simulink model "Adapted_AD9856"  (Simulink 7.6)
settings: Solver=VariableStepDiscrete  StartTime=0.0  StopTime=20000 * SampleTime  RelTol=1e-3
PreLoadFcn:
  | setup_Adapted_AD9856;
InitFcn:
  | setup_Adapted_AD9856;
  | %% DSPBuilder Start
  | alt_dspbuilder_update_model(bdroot)
  | %% DSPBuilder End
values from neighbouring files (symbols this model uses):
  ChanCount = 2    [setup_Adapted_AD9856.m]
  Period = ClockRate / SampleRate    (= 80)    [setup_Adapted_AD9856.m]
  SampleRate = ' num2str(SampleRate) '    [setup_Adapted_AD9856.m]
  SampleTime = ' num2str(SampleTime) ';'])    [setup_Adapted_AD9856.m]
undefined symbols (not defined in the file or in its folder): dpoly, dspba_ChannelInVis, dspba_ChannelOutVis, dspba_internal_get_channel_ports, firhalfband, get, value
libraries: DSPBABase x20, DSPBAPrim x20, allblocks_alteradspbuilder2 x13, simulink x12, DSPBAFilters x5, dspsigops x2, dspsnks4 x2, DSPBAWaveformSynth x1
settings Model: Creator=lkong  LastModifiedBy=akarapet
settings OptimizationCC: InitFltsAndDblsToZero=on
settings DebuggingCC: StrictBusMsg=Warning

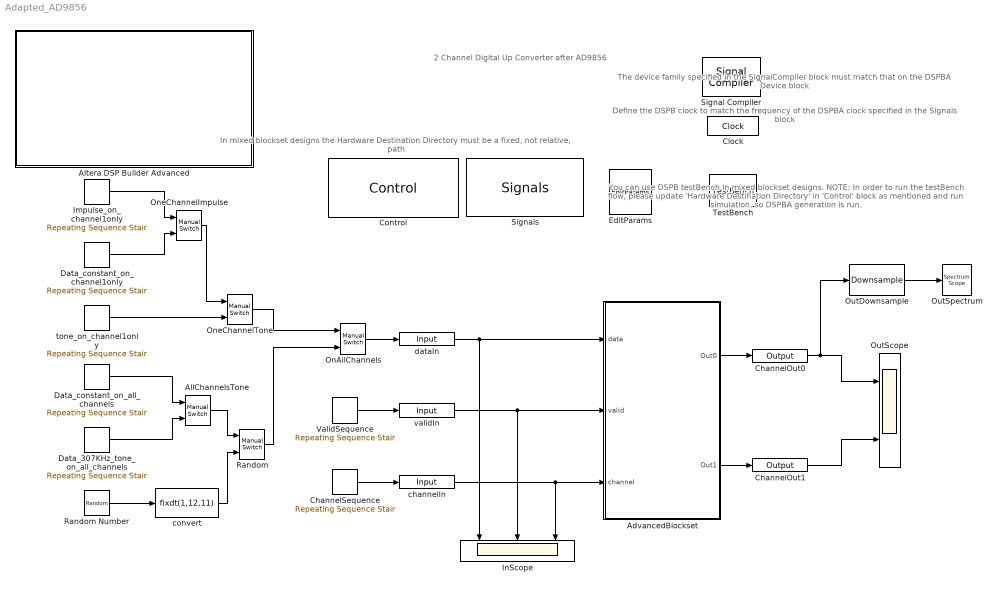
== system Adapted_AD9856 ==
  note: 2 Channel Digital Up Converter after AD9856
  note: In mixed blockset designs the Hardware Destination
      | Directory must be a fixed, not relative, path
  note: Define the DSPB clock to match the frequency of
      | the DSPBA clock specified in the Signals block
  note: You can use DSPB testBench in mixed blockset designs.
      |
      | NOTE: In order to run the testBench flow,  please update
      | 'Hardware Destination Directory' in 'Control' block as mentioned
      | and run simulation, so DSPBA generation is run.
  note: The device family specified in the SignalCompiler
      | block must match that on the DSPBA Device block
  AdvancedBlockset : Subsystem
  AllChannelsTone : simulink/Signal Routing/Manual Switch  SystemSampleTime=-1  sw=0  action=0  varsize=off
  Altera DSP Builder Advanced : Subsystem
      settings: OpenFcn=web('http://www.altera.com', '-new');
      mask Type: DSP Builder Advanced Blockset Ignored Block
      mask Display: image(imread('alteralogo.tif'));
  ChannelOut0 : allblocks_alteradspbuilder2/Output  iofile=/data/akarapet/qshell_linux64_test/p4/dsp_builder/dsp_builder2/Documentation/DesignExamples/Demos/CombinedBlockset/demo_adapted_ad9856/tb_Adapted_AD9856/Adapted%5FAD9856_ChannelOut0.capture  BusType=Signed Fractional  bwl=1  bwr=15  externalType=Inferred  PORTTYPE=Output  allowFloatingPointOverride=on  logOutputs=off
  ChannelOut1 : allblocks_alteradspbuilder2/Output  iofile=/data/akarapet/qshell_linux64_test/p4/dsp_builder/dsp_builder2/Documentation/DesignExamples/Demos/CombinedBlockset/demo_adapted_ad9856/tb_Adapted_AD9856/Adapted%5FAD9856_ChannelOut1.capture  BusType=Signed Fractional  bwl=1  bwr=15  externalType=Inferred  PORTTYPE=Output  allowFloatingPointOverride=on  logOutputs=off
  ChannelSequence : simulink/Sources/Repeating Sequence Stair  SystemSampleTime=-1  OutValues=[[0:ChanCount-1] zeros(1,Period-ChanCount)].'  tsamp=SampleTime  OutMin=[]  OutMax=[]  OutDataTypeStr=fixdt(0,8,0)  OutputDataTypeScalingMode=Specify via dialog  OutDataType=ufix(8)  ConRadixGroup=Use specified scaling  OutScaling=2^-0
  Clock : allblocks_alteradspbuilder2/Clock  ClockPeriod=50  ClockPeriodUnit=ns  SampleTime=1  ResetLatency=0  ResetRegisterCascadeDepth=0  SimulationStartCycle=5  PhaseOffset=0  Reset=aclr  ResetType=Active Low  Export=off
  Control : DSPBABase/Control  generate=on  destination=.  language=VHDL  autotestbench=on  signaldepth=2  coveragetestbench=on  logs=off  spacewidth=2  spacenum=1  addrwidth=12  datawidth=32  dataendian=Big Endian  hierarchicalnames=on  ramThresholdBits=-1  distRamThresholdBits=-1  mlabThresholdBits=-1  hardMultiplierThresholdLuts=-1  version=20090407  errorOnChanMismatch=1  errorOnGPIOMismatch=0  importModelsimResults=0
  Data_307KHz_tone_on_all_channels : simulink/Sources/Repeating Sequence Stair  SystemSampleTime=-1  OutValues="floor([(ChanCount:-1:1)/ChanCount * 1 zeros(1, Period-ChanCount) (ChanCount:-1:1)/ChanCount  * 0 zeros(1, Period-ChanCount) (ChanCount:-1:1)/ChanCount * -1 zeros(1, Period-ChanCount) (ChanCount:-1:1)/ChanCount * 0 zeros(1, Period-ChanCount) ]*1412) / 2^11"  tsamp=SampleTime  OutMin=[]  OutMax=[]  OutDataTypeStr=fixdt(1,12,11)  OutputDataTypeScalingMode=Specify via dialog  OutDataType=sfix(12)  ConRadixGroup=Use specified scaling  OutScaling=2^-11
  Data_constant_on_all_channels : simulink/Sources/Repeating Sequence Stair  SystemSampleTime=-1  OutValues=floor([(ChanCount:-1:1)/ChanCount zeros(1, Period-ChanCount)] * 1412) / 2^11  tsamp=SampleTime  OutMin=[]  OutMax=[]  OutDataTypeStr=fixdt(1,12,11)  OutputDataTypeScalingMode=Specify via dialog  OutDataType=sfix(12)  ConRadixGroup=Use specified scaling  OutScaling=2^-11
  Data_constant_on_channel1only : simulink/Sources/Repeating Sequence Stair  SystemSampleTime=-1  OutValues="[ones(1, 1)  * 1 zeros(1, 199) ]*(1412 / 2^11)"  tsamp=SampleTime  OutMin=[]  OutMax=[]  OutDataTypeStr=fixdt(1,12,11)  OutputDataTypeScalingMode=Specify via dialog  OutDataType=sfix(12)  ConRadixGroup=Use specified scaling  OutScaling=2^-11
  EditParams : DSPBABase/EditParams  SystemSampleTime=-1  version=20090407
  Impulse_on_channel1only : simulink/Sources/Repeating Sequence Stair  SystemSampleTime=-1  OutValues="[ones(1, 1)  * 1 zeros(1, 19900) ]*(1000 / 2^11)"  tsamp=SampleTime  OutMin=[]  OutMax=[]  OutDataTypeStr=fixdt(1,12,11)  OutputDataTypeScalingMode=Specify via dialog  OutDataType=sfix(12)  ConRadixGroup=Use specified scaling  OutScaling=2^-11
  InScope : Scope  NumInputPorts=3
      settings: TimeRange=10000  YMin=-1~-1.5~-1.5  YMax=1~1.5~1.5  SaveName=ScopeData5
  OnAllChannels : simulink/Signal Routing/Manual Switch  SystemSampleTime=-1  sw=0  action=0  varsize=off
  OneChannelImpulse : simulink/Signal Routing/Manual Switch  SystemSampleTime=-1  sw=1  action=0  varsize=off
  OneChannelTone : simulink/Signal Routing/Manual Switch  SystemSampleTime=-1  sw=1  action=0  varsize=off
  OutDownsample : dspsigops/Downsample  N=2  phase=0  InputProcessing=Inherited (this choice will be removed - see release notes)  RateOptions=Enforce single-rate processing  smode=Allow multirate  fmode=Maintain input frame size  ic=0
  OutScope : Scope  NumInputPorts=2
      settings: TimeRange=10000  YMin=-0.75~-1  YMax=0.75~1
  OutSpectrum : dspsnks4/Spectrum Scope  DialogController=dspdialog.SpectrumScope  DialogControllerArgs=DataTag3  SystemSampleTime=-1  ScopeProperties=on  Domain=Frequency  HorizSpan=1  UseBuffer=on  BufferSize=1024  Overlap=0  inpFftLenInherit=off  FFTlength=128  numAvg=9  DisplayProperties=off  AxisGrid=on  Memory=off  FrameNumber=on  AxisLegend=on  AxisZoom=off  OpenScopeAtSimStart=on  OpenScopeImmediately=off  FigPos=get(0,'defaultfigureposition')  AxisProperties=off  XUnits=Hertz  XRange=[0...Fs/2]  XDisplay=0  InheritXIncr=off  XIncr=1/(100e6)  XLabel=Samples  XLimit=Auto  YUnits=dBW/Hertz  XMax=1  XMin=0  YLabel=Magnitude-squared, dB  LineProperties=off  LineDisables=on|off|on|on|on|on|on  LineStyles=-  LineMarkers=None  LineColors=[1 0 1]|[0 0 1]  wintypeSpecScope=Hann  RsSpecScope=50  betaSpecScope=5  winsampSpecScope=Periodic  XAxisParamsVer=6.8
      settings: YMin=-191.5695  YMax=-66.8917
  Random : simulink/Signal Routing/Manual Switch  SystemSampleTime=-1  sw=0  action=0  varsize=off
  Random Number : RandomNumber  SampleTime=SampleTime
  Signal Compiler : allblocks_alteradspbuilder2/Signal Compiler  DeviceFamily=Stratix III  DeviceName=AUTO  EnableSignalTap=off  SignalTapDepth=128  UseBoardBlock=off  StpUseDefaultClock=on  StpClock=Clock  ExportDir=/home/akarapet
  Signals : DSPBABase/Signals  SystemSampleTime=-1  clk=clk  freq=200  margin=0  rst=areset  rstactive=High  bus=bus  enbusclock=on  busfreq=50  bussync=on  version=20090407
  TestBench : allblocks_alteradspbuilder2/TestBench  enable=on  advancedMode=off  modelSimGui=off  maxDisplayErrors=10  mismatchErrorLevel=Error  simdatafile=/data/akarapet/qshell_linux64_test/p4/dsp_builder/dsp_builder2/Documentation/DesignExamples/Demos/CombinedBlockset/demo_adapted_ad9856/tb_Adapted_AD9856/Adapted_AD9856.simdata.tcl
  ValidSequence : simulink/Sources/Repeating Sequence Stair  SystemSampleTime=-1  OutValues=[ones(1,ChanCount) zeros(1,Period-ChanCount)].'  tsamp=SampleTime  OutMin=[]  OutMax=[]  OutDataTypeStr=Inherit: Inherit via back propagation  OutDataType=ufix(1)  ConRadixGroup=Use specified scaling  OutScaling=2^-0
  channelIn : allblocks_alteradspbuilder2/Input  iofile=/data/akarapet/qshell_linux64_test/p4/dsp_builder/dsp_builder2/Documentation/DesignExamples/Demos/CombinedBlockset/demo_adapted_ad9856/tb_Adapted_AD9856/Adapted%5FAD9856_channelIn.salt  BusType=Unsigned Integer  bwl=8  bwr=11  SpecifyClock=off  PORTTYPE=Input  externalType=Inferred  allowFloatingPointOverride=on  logOutputs=off
  convert : DataTypeConversion  OutDataTypeStr=fixdt(1,12,11)
  dataIn : allblocks_alteradspbuilder2/Input  iofile=/data/akarapet/qshell_linux64_test/p4/dsp_builder/dsp_builder2/Documentation/DesignExamples/Demos/CombinedBlockset/demo_adapted_ad9856/tb_Adapted_AD9856/Adapted%5FAD9856_dataIn.salt  BusType=Signed Fractional  bwl=1  bwr=11  SpecifyClock=off  PORTTYPE=Input  externalType=Inferred  allowFloatingPointOverride=on  logOutputs=off
  tone_on_channel1only : simulink/Sources/Repeating Sequence Stair  SystemSampleTime=-1  OutValues="[ones(1, 1)  * 1 zeros(1, Period-1) ones(1, 1)  * 0 zeros(1, Period-1) ones(1, 1)  * -1 zeros(1, Period-1) ones(1, 1)  * 0 zeros(1, Period-1) ]*(1412 / 2^11)"  tsamp=SampleTime  OutMin=[]  OutMax=[]  OutDataTypeStr=fixdt(1,12,11)  OutputDataTypeScalingMode=Specify via dialog  OutDataType=sfix(12)  ConRadixGroup=Use specified scaling  OutScaling=2^-11
  validIn : allblocks_alteradspbuilder2/Input  iofile=/data/akarapet/qshell_linux64_test/p4/dsp_builder/dsp_builder2/Documentation/DesignExamples/Demos/CombinedBlockset/demo_adapted_ad9856/tb_Adapted_AD9856/Adapted%5FAD9856_validIn.salt  BusType=Single Bit  bwl=1  bwr=11  SpecifyClock=off  PORTTYPE=Input  externalType=Inferred  allowFloatingPointOverride=on  logOutputs=off
  wires:
  OnAllChannels/1 -> dataIn/1
  OneChannelTone/1 -> OnAllChannels/1
  Random/1 -> OnAllChannels/2
  Data_constant_on_all_channels/1 -> AllChannelsTone/1
  Data_307KHz_tone_on_all_channels/1 -> AllChannelsTone/2
  tone_on_channel1only/1 -> OneChannelTone/2
  ValidSequence/1 -> validIn/1
  ChannelSequence/1 -> channelIn/1
  OneChannelImpulse/1 -> OneChannelTone/1
  Data_constant_on_channel1only/1 -> OneChannelImpulse/2
  Impulse_on_channel1only/1 -> OneChannelImpulse/1
  OutDownsample/1 -> OutSpectrum/1
  AdvancedBlockset/1(Out0) -> ChannelOut0/1
  AllChannelsTone/1 -> Random/1
  Random Number/1 -> convert/1
  convert/1 -> Random/2
  dataIn/1 -> AdvancedBlockset/1(data), InScope/1
  validIn/1 -> AdvancedBlockset/2(valid), InScope/2
  channelIn/1 -> AdvancedBlockset/3(channel), InScope/3
  ChannelOut0/1 -> OutDownsample/1, OutScope/1
  AdvancedBlockset/2(Out1) -> ChannelOut1/1
  ChannelOut1/1 -> OutScope/2

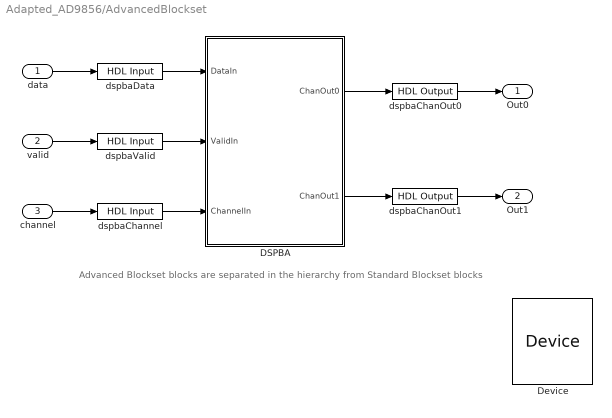
== system Adapted_AD9856/AdvancedBlockset ==
  note: Advanced Blockset blocks are separated in the hierarchy from Standard Blockset blocks
  data : Inport
  valid : Inport  Port=2
  channel : Inport  Port=3
  DSPBA : Subsystem
  Device : DSPBABase/Device  SystemSampleTime=-1  family=Stratix III  stratix4device=Stratix IV E  hardcopy4device=HardCopy IV E  stratix5device=Stratix V GX  device=AUTO  speed=2  stratixSpeed=-5  stratix2Speed=-3  stratix3Speed=-2  stratix4gxSpeed=-2  stratix4gtSpeed=-1  cyclone2Speed=-6  cyclone3Speed=-6  arria2Speed=-4  cyclone4eSpeed=-8  stratix5Speed=-3  arria5Speed=-4  arriaSpeed=-6  cyclone3lsSpeed=-7  cyclone5Speed=-6  arria2gzSpeed=-3  nightFurySpeed=-2  ecp2Speed=-7  hardcopycompat=off  version=20110729
  dspbaChanOut0 : allblocks_alteradspbuilder2/HDL Output  BusType=Signed Fractional  bwl=1  bwr=15  externalType=Inferred
  dspbaChanOut1 : allblocks_alteradspbuilder2/HDL Output  BusType=Signed Fractional  bwl=1  bwr=15  externalType=Inferred
  dspbaChannel : allblocks_alteradspbuilder2/HDL Input  BusType=Unsigned Integer  bwl=8  bwr=0  externalType=Inferred
  dspbaData : allblocks_alteradspbuilder2/HDL Input  BusType=Signed Fractional  bwl=1  bwr=11  externalType=Simulink Fixed Point Type
  dspbaValid : allblocks_alteradspbuilder2/HDL Input  BusType=Single Bit  bwl=8  bwr=0  externalType=Inferred
  Out0 : Outport
  Out1 : Outport  Port=2
  wires:
  DSPBA/1(ChanOut0) -> dspbaChanOut0/1
  data/1 -> dspbaData/1
  valid/1 -> dspbaValid/1
  channel/1 -> dspbaChannel/1
  DSPBA/2(ChanOut1) -> dspbaChanOut1/1
  dspbaData/1 -> DSPBA/1(DataIn)
  dspbaValid/1 -> DSPBA/2(ValidIn)
  dspbaChannel/1 -> DSPBA/3(ChannelIn)
  dspbaChanOut0/1 -> Out0/1
  dspbaChanOut1/1 -> Out1/1

== system Adapted_AD9856/Altera DSP Builder Advanced ==

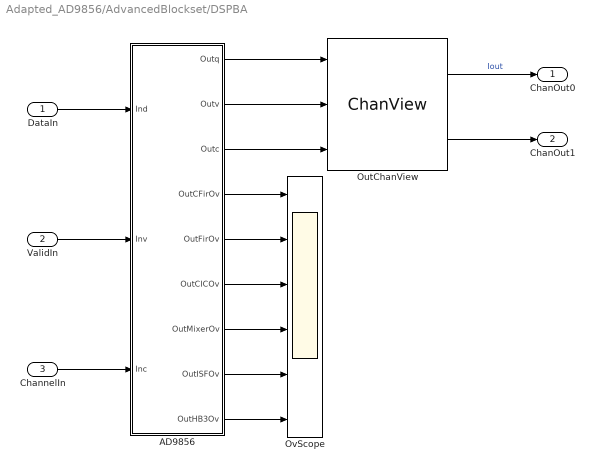
== system Adapted_AD9856/AdvancedBlockset/DSPBA ==
  DataIn : Inport
  ValidIn : Inport  Port=2
  ChannelIn : Inport  Port=3
  AD9856 : Subsystem
  OutChanView : DSPBABase/ChanView  nchans=2  chan_vector=[0 1]  outsvalid=off  latency=2  version=20090407
  OvScope : Scope  NumInputPorts=6
      settings: TimeRange=5e-005  YMin=-1~-1~-1~-1~-1~-5  YMax=1~1~1~1~1~5  SaveName=ScopeData4
  ChanOut0 : Outport
  ChanOut1 : Outport  Port=2
  wires:
  AD9856/1(Outq) -> OutChanView/1
  AD9856/2(Outv) -> OutChanView/2
  AD9856/3(Outc) -> OutChanView/3
  AD9856/4(OutCFirOv) -> OvScope/1
  AD9856/5(OutFirOv) -> OvScope/2
  AD9856/6(OutCICOv) -> OvScope/3
  AD9856/7(OutMixerOv) -> OvScope/4
  AD9856/8(OutISFOv) -> OvScope/5
  AD9856/9(OutHB3Ov) -> OvScope/6
  OutChanView/1 -> ChanOut0/1  "Iout"
  DataIn/1 -> AD9856/1(Ind)
  OutChanView/2 -> ChanOut1/1
  ValidIn/1 -> AD9856/2(Inv)
  ChannelIn/1 -> AD9856/3(Inc)

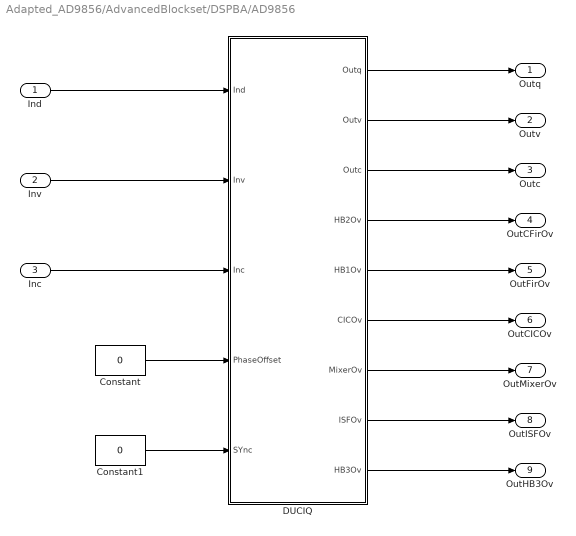
== system Adapted_AD9856/AdvancedBlockset/DSPBA/AD9856 ==
  Ind : Inport
  Inv : Inport  Port=2
  Inc : Inport  Port=3
  Constant : Constant  Value=0  OutDataTypeStr=Inherit: Inherit via back propagation  SampleTime=SampleTime
  Constant1 : Constant  Value=0  OutDataTypeStr=Inherit: Inherit via back propagation  SampleTime=SampleTime
  DUCIQ : Subsystem
  Outq : Outport
  Outv : Outport  Port=2
  Outc : Outport  Port=3
  OutCFirOv : Outport  Port=4
  OutFirOv : Outport  Port=5
  OutCICOv : Outport  Port=6
  OutMixerOv : Outport  Port=7
  OutISFOv : Outport  Port=8
  OutHB3Ov : Outport  Port=9
  wires:
  DUCIQ/1(Outq) -> Outq/1
  Ind/1 -> DUCIQ/1(Ind)
  DUCIQ/2(Outv) -> Outv/1
  Inv/1 -> DUCIQ/2(Inv)
  DUCIQ/3(Outc) -> Outc/1
  Inc/1 -> DUCIQ/3(Inc)
  DUCIQ/4(HB2Ov) -> OutCFirOv/1
  DUCIQ/5(HB1Ov) -> OutFirOv/1
  Constant/1 -> DUCIQ/4(PhaseOffset)
  DUCIQ/6(CICOv) -> OutCICOv/1
  Constant1/1 -> DUCIQ/5(SYnc)
  DUCIQ/8(ISFOv) -> OutISFOv/1
  DUCIQ/9(HB3Ov) -> OutHB3Ov/1
  DUCIQ/7(MixerOv) -> OutMixerOv/1

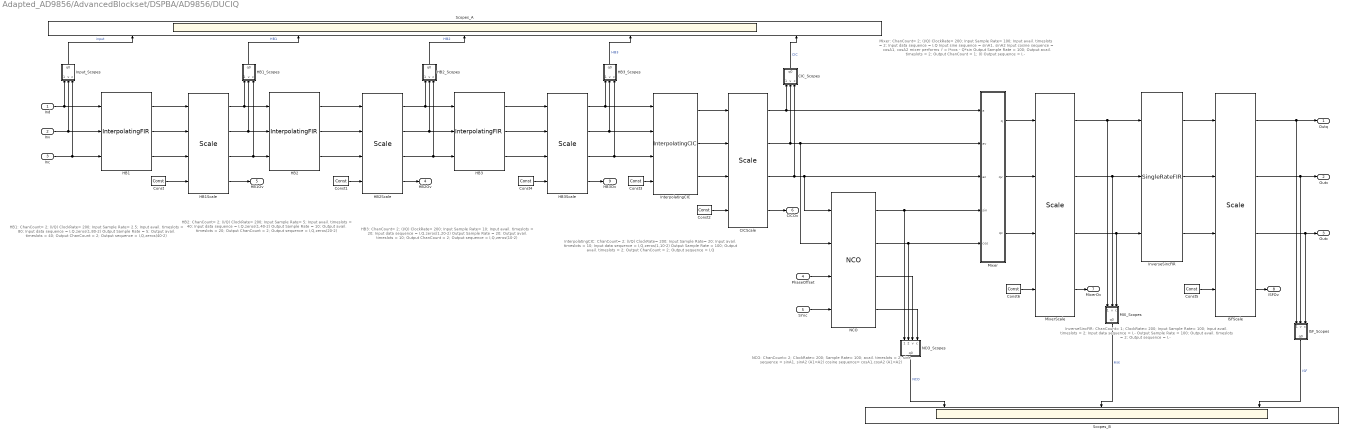
== system Adapted_AD9856/AdvancedBlockset/DSPBA/AD9856/DUCIQ ==
  note: HB1:
      | ChanCount= 2; (I/Q)
      | ClockRate= 200;
      | Input Sample Rate= 2.5;
      | Input avail. timeslots = 80;
      | Input data sequence = I,Q,zeros(1,80-2)
      | Output Sample Rate = 5;
      | Output avail. timeslots = 40;
      | Output ChanCount = 2;
      | Output sequence = I,Q,zeros(40-2)
  note: HB2:
      | ChanCount= 2; (I/Q)
      | ClockRate= 200;
      | Input Sample Rate= 5;
      | Input avail. timeslots = 40;
      | Input data sequence = I,Q,zeros(1,40-2)
      | Output Sample Rate = 10;
      | Output avail. timeslots = 20;
      | Output ChanCount = 2;
      | Output sequence = I,Q,zeros(20-2)
  note: HB3:
      | ChanCount= 2; (I/Q)
      | ClockRate= 200;
      | Input Sample Rate= 10;
      | Input avail. timeslots = 20;
      | Input data sequence = I,Q,zeros(1,20-2)
      | Output Sample Rate = 20;
      | Output avail. timeslots = 10;
      | Output ChanCount = 2;
      | Output sequence = I,Q,zeros(10-2)
  note: InterpolatingCIC:
      | ChanCount= 2; (I/Q)
      | ClockRate= 200;
      | Input Sample Rate= 20;
      | Input avail. timeslots = 10;
      | Input data sequence = I,Q,zeros(1,10-2)
      | Output Sample Rate = 100;
      | Output avail. timeslots = 2;
      | Output ChanCount = 2;
      | Output sequence = I,Q
  note: NCO:
      | ChanCount= 2;
      | ClockRate= 200;
      | Sample Rate= 100;
      | avail. timeslots = 2;
      | sine sequence = sinA1, sinA2 (A1=A2)
      | cosine sequence= cosA1,cosA2 (A1=A2)
  note: Mixer:
      | ChanCount= 2; (I/Q)
      | ClockRate= 200;
      | Input Sample Rate= 100;
      | Input avail. timeslots = 2;
      | Input data sequence = I,Q
      | Input sine sequence = sinA1, sinA2
      | Input cosine sequence = cosA1, cosA2
      | mixer performs i' = I*cos - Q*sin
      | Output Sample Rate = 100;
      | Output avail. timeslots = 2;
      | Output ChanCount = 1; (I)
      | Output sequence = I,-
  note: InverseSincFIR:
      | ChanCount= 1;
      | ClockRate= 200;
      | Input Sample Rate= 100;
      | Input avail. timeslots = 2;
      | Input data sequence = I,-
      | Output Sample Rate = 100;
      | Output avail. timeslots = 2;
      | Output sequence = I,-
  Ind : Inport
  Inv : Inport  Port=2
  Inc : Inport  Port=3
  PhaseOffset : Inport  Port=4
  SYnc : Inport  Port=5
  CICScale : DSPBABase/Scale  otype=sfix(16)  scale=2^-15  rndmethod=Unbiased  factor=1  satmethod=Symmetric  shift_vec=[-7 -8]  latency=5  version=20090407
  CIC_Scopes : Subsystem
  Const{,1..2,4..6} (6 alike) : DSPBAPrim/Const  primtype=const  nInputs=0  nOutputs=1  omode=Specify via dialog  otype=ufix(1)  scale=2^-0  rndmethod=Unbiased  factor=1  satmethod=Symmetric  shift_vec=[0 1 2 -1]  value=0  inPortNames=['+'; '+';]  outPortNames=[' ']  dspbaimage=dspba_prim.jpg  text=fprintf('%g', value);  style=Optimised  visibilities=8 + 1024  floatPrecision=float32_m23  version=20120820
  Const3 : DSPBAPrim/Const  primtype=const  nInputs=0  nOutputs=1  omode=boolean  otype=sfix(16)  scale=2^-15  rndmethod=Unbiased  factor=1  satmethod=Symmetric  shift_vec=[0 1 2 -1]  value=0  inPortNames=['+'; '+';]  outPortNames=[' ']  dspbaimage=dspba_prim.jpg  text=fprintf('%g', value);  style=Optimised  visibilities=8 + 1024  floatPrecision=float32_m23  version=20120820
  HB1 : DSPBAFilters/InterpolatingFIR  nInputRate=SampleRate  interp=2  nchan=2  symmetry=Symmetrical  coef=fi(firhalfband(46, 0.35 ),1,16,15)  addr=512  rwmode=Read/Write  nband=Use All Taps  exposebus=off  latency=34  version=20090407
  HB1Scale : DSPBABase/Scale  otype=sfix(16)  scale=2^-15  rndmethod=Unbiased  factor=1  satmethod=Symmetric  shift_vec=0  latency=3  version=20090407
  HB1_Scopes : Subsystem
  HB2 : DSPBAFilters/InterpolatingFIR  nInputRate=SampleRate * 2  interp=2  nchan=2  symmetry=Symmetrical  coef=fi(firhalfband(38, 0.25 ),1,16,15)  addr=1024  rwmode=Read/Write  nband=Use All Taps  exposebus=off  latency=30  version=20090407
  HB2Scale : DSPBABase/Scale  otype=sfix(16)  scale=2^-15  rndmethod=Unbiased  factor=1  satmethod=Symmetric  shift_vec=[1 1]  latency=5  version=20090407
  HB2_Scopes : Subsystem
  HB3 : DSPBAFilters/InterpolatingFIR  nInputRate=SampleRate * 4  interp=2  nchan=2  symmetry=Symmetrical  coef=fi(firhalfband(18, 0.21 ),1,16,15)  addr=1536  rwmode=Read/Write  nband=Use All Taps  exposebus=off  latency=20  version=20090407
  HB3Scale : DSPBABase/Scale  otype=sfix(16)  scale=2^-15  rndmethod=Unbiased  factor=1  satmethod=Symmetric  shift_vec=[1 1]  latency=5  version=20090407
  HB3_Scopes : Subsystem
  ISFScale : DSPBABase/Scale  otype=sfix(16)  scale=2^-15  rndmethod=Unbiased  factor=1  satmethod=Symmetric  shift_vec=0  latency=3  version=20090407
  ISF_Scopes : Subsystem
  Input_Scopes : Subsystem
  InterpolatingCIC : DSPBAFilters/InterpolatingCIC  nInputRate=SampleRate * 8  nchan=2  nstages=4  nrate=5  ndelay=1  ndecimation=1  sHints='*delay* arch mem'  inWidth=1  outWidth=1  sysClock=200  latency=9  version=20090407
  InverseSincFIR : DSPBAFilters/SingleRateFIR  nInputRate=SampleRate * 40  nchan=1  symmetry=Symmetrical  coef=fi(fir1(16, 0.7),1,16,15)  addr=2048  rwmode=Read/Write  nband=Use All Taps  latency=13  exposebus=off  version=20090407
  MIX_Scopes : Subsystem
  Mixer : Subsystem
  MixerScale : DSPBABase/Scale  otype=sfix(16)  scale=2^-15  rndmethod=Unbiased  factor=1  satmethod=Symmetric  shift_vec=[0]  latency=3  version=20090407
  NCO : DSPBAWaveformSynth/NCO  outputRate=SampleRate * 40  otype=sfix(18)  scale=2^-17  expSFDR=108.36  accumBitWidth=30  accumPrecision=+/- 0.046566  phaseIncrAndInv=[0.61 0.61] * 2^30 /6.144  phaseIncrInMHz="[9.92839  9.92839]"  phaseIncrAndInvMap=2046  rwmode=Read/Write  exposebus=off  outWidth=1  tableSize=8  latency=14  version=20090407
  NCO_Scopes : Subsystem
  Scopes_A : Scope  NumInputPorts=5
      settings: TimeRange=5e-005  YMin=-1~-1~-1~-1~-0.75  YMax=1~0.75~0.75~0.75~0.75
  Scopes_B : Scope  NumInputPorts=3
      settings: TimeRange=5e-005  YMin=-1~-1~-1  YMax=1~1~1  SaveName=ScopeData2
  Outq : Outport
  Outv : Outport  Port=2
  Outc : Outport  Port=3
  HB2Ov : Outport  Port=4
  HB1Ov : Outport  Port=5
  CICOv : Outport  Port=6
  MixerOv : Outport  Port=7
  ISFOv : Outport  Port=8
  HB3Ov : Outport  Port=9
  wires:
  HB1/1 -> HB1Scale/1
  HB1/2 -> HB1Scale/2
  HB1/3 -> HB1Scale/3
  HB1Scale/1 -> HB2/1, HB1_Scopes/1(d0)
  HB1Scale/2 -> HB2/2, HB1_Scopes/2(v)
  HB1Scale/3 -> HB2/3, HB1_Scopes/3(c)
  HB2/1 -> HB2Scale/1
  HB2/2 -> HB2Scale/2
  HB2/3 -> HB2Scale/3
  HB2Scale/1 -> HB3/1, HB2_Scopes/1(d0)
  HB2Scale/2 -> HB3/2, HB2_Scopes/2(v)
  HB2Scale/3 -> HB3/3, HB2_Scopes/3(c)
  NCO/1 -> NCO_Scopes/1(sin0), Mixer/4(sin)
  NCO/2 -> NCO_Scopes/2(cos0), Mixer/5(cos)
  CICScale/1 -> CIC_Scopes/1(d0), Mixer/1(a)
  CICScale/2 -> NCO/2, Mixer/2(av), CIC_Scopes/2(v)
  CICScale/3 -> NCO/1, Mixer/3(ac), CIC_Scopes/3(c)
  InterpolatingCIC/1 -> CICScale/1
  InterpolatingCIC/2 -> CICScale/2
  InterpolatingCIC/3 -> CICScale/3
  Const/1 -> HB1Scale/4
  Const1/1 -> HB2Scale/4
  Const2/1 -> CICScale/4
  Const3/1 -> InterpolatingCIC/4
  Ind/1 -> HB1/1, Input_Scopes/1(d0)
  Inv/1 -> HB1/2, Input_Scopes/2(v)
  Inc/1 -> HB1/3, Input_Scopes/3(c)
  PhaseOffset/1 -> NCO/3
  SYnc/1 -> NCO/4
  HB2Scale/4 -> HB2Ov/1
  HB1Scale/4 -> HB1Ov/1
  CICScale/4 -> CICOv/1
  NCO/3 -> NCO_Scopes/3(v)
  NCO/4 -> NCO_Scopes/4(c)
  Input_Scopes/1(q0) -> Scopes_A/1  "input"
  HB1_Scopes/1(q0) -> Scopes_A/2  "HB1"
  HB2_Scopes/1(q0) -> Scopes_A/3  "HB2"
  CIC_Scopes/1(q0) -> Scopes_A/5  "CIC"
  NCO_Scopes/1(q0) -> Scopes_B/1  "NCO"
  MIX_Scopes/1(q0) -> Scopes_B/2  "MIX"
  ISF_Scopes/1(q0) -> Scopes_B/3  "ISF"
  HB3/1 -> HB3Scale/1
  HB3/2 -> HB3Scale/2
  HB3/3 -> HB3Scale/3
  HB3Scale/1 -> InterpolatingCIC/1, HB3_Scopes/1(d0)
  HB3Scale/2 -> InterpolatingCIC/2, HB3_Scopes/2(v)
  HB3Scale/3 -> InterpolatingCIC/3, HB3_Scopes/3(c)
  Const4/1 -> HB3Scale/4
  HB3Scale/4 -> HB3Ov/1
  HB3_Scopes/1(q0) -> Scopes_A/4  "HB3"
  Mixer/1(q) -> MixerScale/1
  Mixer/2(qv) -> MixerScale/2
  Mixer/3(qc) -> MixerScale/3
  MixerScale/2 -> MIX_Scopes/2(v), InverseSincFIR/2
  MixerScale/3 -> MIX_Scopes/3(c), InverseSincFIR/3
  Const6/1 -> MixerScale/4
  MixerScale/4 -> MixerOv/1
  ISFScale/1 -> Outq/1, ISF_Scopes/1(d0)
  ISFScale/2 -> Outv/1, ISF_Scopes/2(v)
  ISFScale/3 -> Outc/1, ISF_Scopes/3(c)
  ISFScale/4 -> ISFOv/1
  Const5/1 -> ISFScale/4
  InverseSincFIR/3 -> ISFScale/3
  InverseSincFIR/2 -> ISFScale/2
  InverseSincFIR/1 -> ISFScale/1
  MixerScale/1 -> MIX_Scopes/1(d0), InverseSincFIR/1

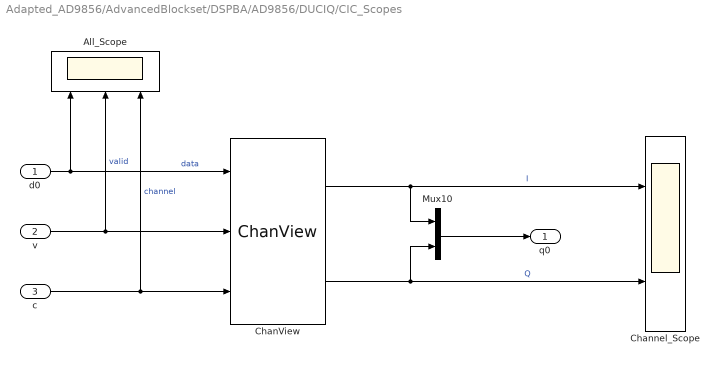
== system Adapted_AD9856/AdvancedBlockset/DSPBA/AD9856/DUCIQ/CIC_Scopes ==
  d0 : Inport
  v : Inport  Port=2
  c : Inport  Port=3
  All_Scope : Scope  NumInputPorts=3
      settings: TimeRange=10000  YMin=-0.125~0~0  YMax=0.125~1~1  SaveName=ScopeData29
  ChanView : DSPBABase/ChanView  nchans=16  chan_vector=[0 1]  outsvalid=off  latency=2  version=20090407
  Channel_Scope : Scope  NumInputPorts=2
      settings: TimeRange=10000  YMin=-0.125~-0.075  YMax=0.125~0.075  SaveName=chanFiltData  DataFormat=Array
  Mux10 : Mux  Inputs=2
  q0 : Outport
  wires:
  d0/1 -> All_Scope/1, ChanView/1  "data"
  v/1 -> All_Scope/2, ChanView/2  "valid"
  c/1 -> All_Scope/3, ChanView/3  "channel"
  ChanView/2 -> Channel_Scope/2, Mux10/2  "Q"
  Mux10/1 -> q0/1
  ChanView/1 -> Channel_Scope/1, Mux10/1  "I"

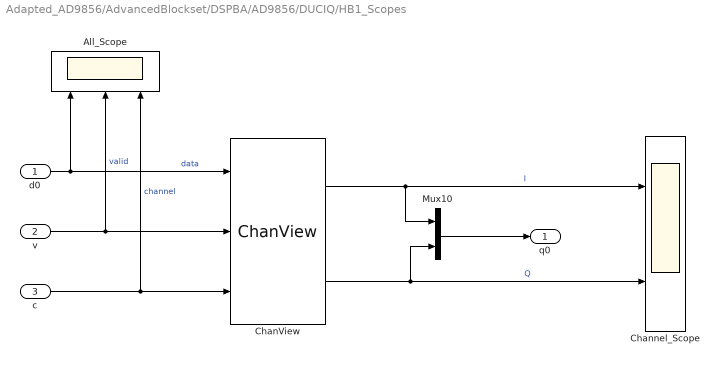
== system Adapted_AD9856/AdvancedBlockset/DSPBA/AD9856/DUCIQ/HB1_Scopes ==
  d0 : Inport
  v : Inport  Port=2
  c : Inport  Port=3
  All_Scope : Scope  NumInputPorts=3
      settings: TimeRange=10000  YMin=-0.125~0~0  YMax=0.125~1~1  SaveName=ScopeData29
  ChanView : DSPBABase/ChanView  nchans=16  chan_vector=[0 1]  outsvalid=off  latency=2  version=20090407
  Channel_Scope : Scope  NumInputPorts=2
      settings: TimeRange=10000  YMin=-0.125~-0.075  YMax=0.125~0.075  SaveName=chanFiltData  DataFormat=Array
  Mux10 : Mux  Inputs=2
  q0 : Outport
  wires:
  Mux10/1 -> q0/1
  ChanView/2 -> Mux10/2, Channel_Scope/2  "Q"
  c/1 -> ChanView/3, All_Scope/3  "channel"
  v/1 -> ChanView/2, All_Scope/2  "valid"
  d0/1 -> ChanView/1, All_Scope/1  "data"
  ChanView/1 -> Channel_Scope/1, Mux10/1  "I"

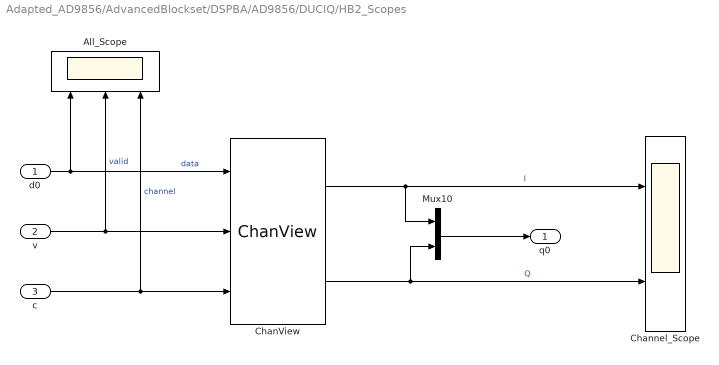
== system Adapted_AD9856/AdvancedBlockset/DSPBA/AD9856/DUCIQ/HB2_Scopes ==
  d0 : Inport
  v : Inport  Port=2
  c : Inport  Port=3
  All_Scope : Scope  NumInputPorts=3
      settings: TimeRange=10000  YMin=-0.125~0~0  YMax=0.125~1~1  SaveName=ScopeData29
  ChanView : DSPBABase/ChanView  nchans=16  chan_vector=[0 1]  outsvalid=off  latency=2  version=20090407
  Channel_Scope : Scope  NumInputPorts=2
      settings: TimeRange=10000  YMin=-0.125~-0.075  YMax=0.125~0.075  SaveName=chanFiltData  DataFormat=Array
  Mux10 : Mux  Inputs=2
  q0 : Outport
  wires:
  d0/1 -> All_Scope/1, ChanView/1  "data"
  v/1 -> All_Scope/2, ChanView/2  "valid"
  c/1 -> All_Scope/3, ChanView/3  "channel"
  ChanView/2 -> Channel_Scope/2, Mux10/2  "Q"
  Mux10/1 -> q0/1
  ChanView/1 -> Mux10/1, Channel_Scope/1  "I"

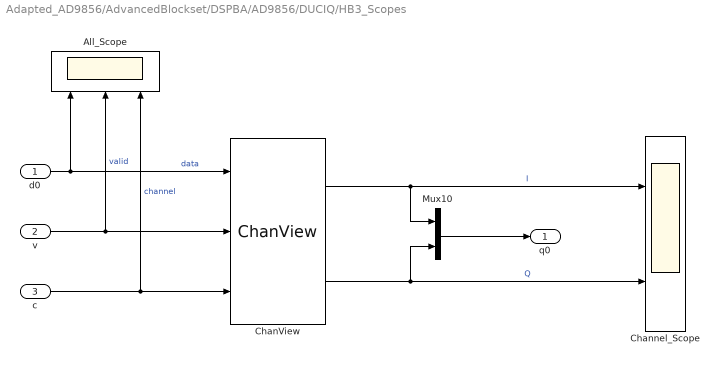
== system Adapted_AD9856/AdvancedBlockset/DSPBA/AD9856/DUCIQ/HB3_Scopes ==
  d0 : Inport
  v : Inport  Port=2
  c : Inport  Port=3
  All_Scope : Scope  NumInputPorts=3
      settings: TimeRange=10000  YMin=-0.125~0~0  YMax=0.125~1~1  SaveName=ScopeData29
  ChanView : DSPBABase/ChanView  nchans=16  chan_vector=[0 1]  outsvalid=off  latency=2  version=20090407
  Channel_Scope : Scope  NumInputPorts=2
      settings: TimeRange=10000  YMin=-0.125~-0.075  YMax=0.125~0.075  SaveName=chanFiltData  DataFormat=Array
  Mux10 : Mux  Inputs=2
  q0 : Outport
  wires:
  Mux10/1 -> q0/1
  ChanView/2 -> Mux10/2, Channel_Scope/2  "Q"
  ChanView/1 -> Channel_Scope/1, Mux10/1  "I"
  c/1 -> ChanView/3, All_Scope/3  "channel"
  v/1 -> ChanView/2, All_Scope/2  "valid"
  d0/1 -> ChanView/1, All_Scope/1  "data"

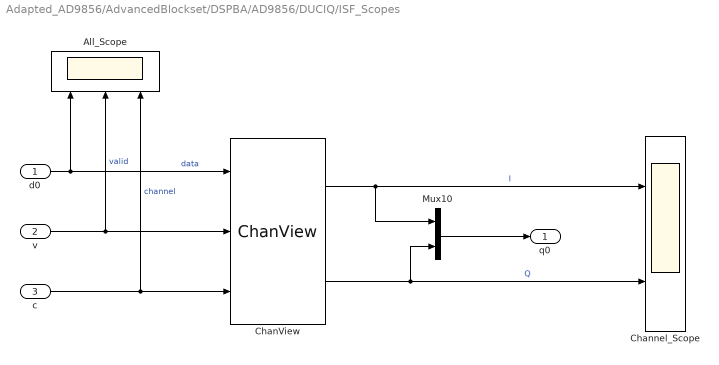
== system Adapted_AD9856/AdvancedBlockset/DSPBA/AD9856/DUCIQ/ISF_Scopes ==
  d0 : Inport
  v : Inport  Port=2
  c : Inport  Port=3
  All_Scope : Scope  NumInputPorts=3
      settings: TimeRange=10000  YMin=-0.125~0~0  YMax=0.125~1~1  SaveName=ScopeData29
  ChanView : DSPBABase/ChanView  nchans=16  chan_vector=[0 1]  outsvalid=off  latency=2  version=20090407
  Channel_Scope : Scope  NumInputPorts=2
      settings: TimeRange=10000  YMin=-0.125~-0.075  YMax=0.125~0.075  SaveName=chanFiltData  DataFormat=Array
  Mux10 : Mux  Inputs=2
  q0 : Outport
  wires:
  d0/1 -> All_Scope/1, ChanView/1  "data"
  v/1 -> All_Scope/2, ChanView/2  "valid"
  c/1 -> All_Scope/3, ChanView/3  "channel"
  ChanView/2 -> Channel_Scope/2, Mux10/2  "Q"
  Mux10/1 -> q0/1
  ChanView/1 -> Mux10/1, Channel_Scope/1  "I"

== system Adapted_AD9856/AdvancedBlockset/DSPBA/AD9856/DUCIQ/Input_Scopes ==
  d0 : Inport
  v : Inport  Port=2
  c : Inport  Port=3
  All_Scope : Scope  NumInputPorts=3
      settings: TimeRange=10000  YMin=-0.125~0~0  YMax=0.125~1~1  SaveName=ScopeData29
  ChanView : DSPBABase/ChanView  nchans=16  chan_vector=[0 1]  outsvalid=off  latency=2  version=20090407
  Channel_Scope : Scope  NumInputPorts=2
      settings: TimeRange=10000  YMin=-0.125~-0.075  YMax=0.125~0.075  SaveName=chanFiltData  DataFormat=Array
  Mux10 : Mux  Inputs=2
  q0 : Outport
  wires:
  d0/1 -> All_Scope/1, ChanView/1  "data"
  v/1 -> All_Scope/2, ChanView/2  "valid"
  c/1 -> All_Scope/3, ChanView/3  "channel"
  ChanView/1 -> Channel_Scope/1, Mux10/1  "I"
  ChanView/2 -> Channel_Scope/2, Mux10/2  "Q"
  Mux10/1 -> q0/1

== system Adapted_AD9856/AdvancedBlockset/DSPBA/AD9856/DUCIQ/MIX_Scopes ==
  d0 : Inport
  v : Inport  Port=2
  c : Inport  Port=3
  All_Scope : Scope  NumInputPorts=3
      settings: TimeRange=0.0005  YMin=-0.25~0~0  YMax=0.225~1~1  SaveName=ScopeData29
  ChanView : DSPBABase/ChanView  nchans=16  chan_vector=[0 1]  outsvalid=off  latency=2  version=20090407
  Channel_Scope : Scope  NumInputPorts=2
      settings: TimeRange=10000  YMin=-0.125~-0.075  YMax=0.125~0.075  SaveName=chanFiltData  DataFormat=Array
  Mux10 : Mux  Inputs=2
  q0 : Outport
  wires:
  Mux10/1 -> q0/1
  ChanView/2 -> Mux10/2, Channel_Scope/2  "Q"
  ChanView/1 -> Mux10/1, Channel_Scope/1  "I"
  c/1 -> ChanView/3, All_Scope/3  "channel"
  v/1 -> ChanView/2, All_Scope/2  "valid"
  d0/1 -> ChanView/1, All_Scope/1  "data"

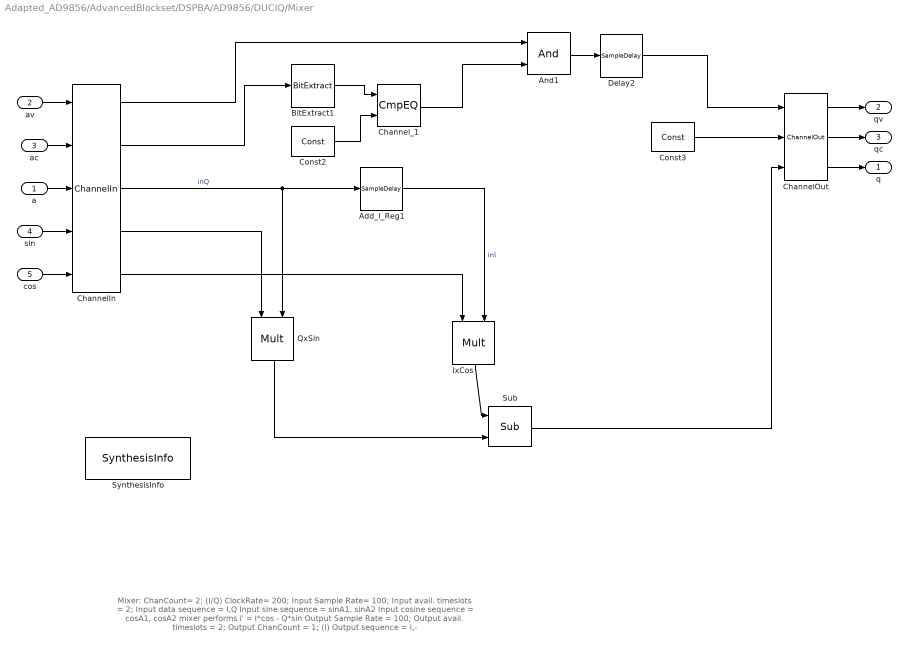
== system Adapted_AD9856/AdvancedBlockset/DSPBA/AD9856/DUCIQ/Mixer ==
  note: Mixer:
      | ChanCount= 2; (I/Q)
      | ClockRate= 200;
      | Input Sample Rate= 100;
      | Input avail. timeslots = 2;
      | Input data sequence = I,Q
      | Input sine sequence = sinA1, sinA2
      | Input cosine sequence = cosA1, cosA2
      | mixer performs i' = I*cos - Q*sin
      | Output Sample Rate = 100;
      | Output avail. timeslots = 2;
      | Output ChanCount = 1; (I)
      | Output sequence = I,-
  a : Inport
  av : Inport  Port=2
  ac : Inport  Port=3
  sin : Inport  Port=4
  cos : Inport  Port=5
  Add_I_Reg1 : DSPBAPrim/SampleDelay  primtype=delay  nInputs=1  nOutputs=1  omode=Inherit via internal rule  otype=sfix(16)  scale=2^-15  rndmethod=Unbiased  factor=1  satmethod=Symmetric  shift_vec=[0 1 2 -1]  value=1  inPortNames=[' '; ' ';]  outPortNames=[' ']  dspbaimage=dspba_prim.jpg  text=dpoly(1, eye(1,value+1), 'z')  style=Optimised  visibilities=8 + 1024  flexible=off  slackgroup=0  augmented=0  version=20090407
  And1 : DSPBAPrim/And  primtype=and  nInputs=2  nOutputs=1  omode=Inherit via internal rule  otype=sfix(16)  scale=2^-15  rndmethod=Unbiased  factor=1  satmethod=Symmetric  shift_vec=[0 1 2 -1]  value=0  inPortNames=[' '; ' ';]  outPortNames=[' ']  dspbaimage=dspba_prim.jpg  text=fprintf('&');  style=Optimised  visibilities=8  version=20090407
  BitExtract1 : DSPBAPrim/BitExtract  primtype=bitextract  nInputs=1  nOutputs=1  omode=Specify via dialog  otype=ufix(2)  scale=2^-0  rndmethod=Unbiased  factor=1  satmethod=Symmetric  shift_vec=[0 1 2 -1]  value=0  inPortNames=[' '; ' ';]  outPortNames=[' ']  dspbaimage=dspba_prim.jpg  text=fprintf('..%d', value);  style=Optimised  visibilities=8 + 1024  version=20090407
  ChannelIn : DSPBAPrim/ChannelIn  primtype=channelin  nInputs=dspba_internal_get_channel_ports(gcb)  nOutputs=dspba_internal_get_channel_ports(gcb)  omode=Inherit via internal rule  otype=sfix(16)  scale=2^-15  rndmethod=Unbiased  factor=1  satmethod=Symmetric  shift_vec=[0 1 2 -1]  value=3  inPortNames=['v'; 'c'; '0'; '1'; '2'; '3'; '4'; '5'; '6'; '7'; '8']  outPortNames=['v'; 'c'; '0'; '1'; '2'; '3'; '4'; '5'; '6'; '7'; '8']  dspbaimage=dspba_prim.jpg  text=fprintf('In');  style=Optimised  dataSignals=3  foldingEnabled=off  channels=1  sampleRate=200  visibilities=dspba_ChannelInVis(gcb)  latencyCorrection=0  version=20090408
  ChannelOut : DSPBAPrim/ChannelOut  primtype=channelout  nInputs=dspba_internal_get_channel_ports(gcb)  nOutputs=dspba_internal_get_channel_ports(gcb)  omode=Inherit via internal rule  otype=sfix(16)  scale=2^-15  rndmethod=Unbiased  factor=1  satmethod=Symmetric  shift_vec=[0 1 2 -1]  value=1  inPortNames=['v'; 'c'; '0'; '1'; '2'; '3'; '4'; '5'; '6'; '7'; '8']  outPortNames=['v'; 'c'; '0'; '1'; '2'; '3'; '4'; '5'; '6'; '7'; '8']  dspbaimage=dspba_prim.jpg  text=fprintf('Out');  style=Optimised  dataSignals=1  foldingEnabled=off  channels=1  sampleRate=200  visibilities=dspba_ChannelOutVis(gcb)  latency=4  latencyCorrection=0  version=20090408
  Channel_1 : DSPBAPrim/CmpEQ  primtype=cmpeq  nInputs=2  nOutputs=1  omode=boolean  otype=sfix(16)  scale=2^-15  rndmethod=Unbiased  factor=1  satmethod=Symmetric  shift_vec=[0 1 2 -1]  value=0  inPortNames=[' '; ' ';]  outPortNames=[' ']  dspbaimage=dspba_prim.jpg  text=fprintf('==');  style=Optimised  visibilities=0  advOptions=[]  version=20130117
  Const2 : DSPBAPrim/Const  primtype=const  nInputs=0  nOutputs=1  omode=Inherit via internal rule  otype=sfix(16)  scale=2^-15  rndmethod=Unbiased  factor=1  satmethod=Symmetric  shift_vec=[0 1 2 -1]  value=0  inPortNames=['+'; '+';]  outPortNames=[' ']  dspbaimage=dspba_prim.jpg  text=fprintf('%g', value);  style=Optimised  visibilities=8 + 1024  floatPrecision=float32_m23  version=20120820
  Const3 : DSPBAPrim/Const  primtype=const  nInputs=0  nOutputs=1  omode=Specify via dialog  otype=uint(8)  scale=2^-15  rndmethod=Unbiased  factor=1  satmethod=Symmetric  shift_vec=[0 1 2 -1]  value=0  inPortNames=['+'; '+';]  outPortNames=[' ']  dspbaimage=dspba_prim.jpg  text=fprintf('%g', value);  style=Optimised  visibilities=8 + 1024  floatPrecision=float32_m23  version=20120820
  Delay2 : DSPBAPrim/SampleDelay  primtype=sampdelay  nInputs=1  nOutputs=1  omode=Inherit via internal rule  otype=sfix(16)  scale=2^-15  rndmethod=Unbiased  factor=1  satmethod=Symmetric  shift_vec=[0 1 2 -1]  value=1  inPortNames=[' '; ' ';]  outPortNames=[' ']  dspbaimage=dspba_prim.jpg  text=dpoly(1, eye(1,value+1), 'z')  style=Optimised  visibilities=8 + 1024  flexible=off  slackgroup=0  augmented=0  version=20090407
  IxCos : DSPBAPrim/Mult  primtype=mult  nInputs=2  nOutputs=1  omode=Inherit via internal rule  otype=sfix(16)  scale=2^-15  rndmethod=Unbiased  factor=1  satmethod=Symmetric  shift_vec=[0 1 2 -1]  value=0  inPortNames=[' '; ' ';]  outPortNames=[' ']  dspbaimage=dspba_prim.jpg  text=fprintf('X');  style=Optimised  visibilities=8  floatPrecision=float32_m23  floatRounding=correct  advOptions=[]  version=20130115
  QxSin : DSPBAPrim/Mult  primtype=mult  nInputs=2  nOutputs=1  omode=Inherit via internal rule  otype=sfix(16)  scale=2^-15  rndmethod=Unbiased  factor=1  satmethod=Symmetric  shift_vec=[0 1 2 -1]  value=0  inPortNames=[' '; ' ';]  outPortNames=[' ']  dspbaimage=dspba_prim.jpg  text=fprintf('X');  style=Optimised  visibilities=8  floatPrecision=float32_m23  floatRounding=correct  advOptions=[]  version=20130115
  Sub : DSPBAPrim/Sub  primtype=sub  nInputs=2  nOutputs=1  omode=Inherit via internal rule with word growth  otype=sfix(16)  scale=2^-15  rndmethod=Unbiased  factor=1  satmethod=Symmetric  shift_vec=[0 1 2 -1]  value=0  inPortNames=['+'; '-';]  outPortNames=[' ']  dspbaimage=dspba_prim.jpg  text=fprintf('-');  style=Optimised  visibilities=8  floatRounding=correct  advOptions=[]  version=20130115
  SynthesisInfo : DSPBAPrim/SynthesisInfo  primtype=synthinfo  nInputs=0  nOutputs=0  omode=Inherit via internal rule  otype=sfix(16)  scale=2^-15  rndmethod=Truncate  factor=1  satmethod=Symmetric  shift_vec=[0 1 2 -1]  value=6  inPortNames=[' '; ' ';]  outPortNames=[' ']  dspbaimage=dspba_prim_ctrl.jpg  text=fprintf('Synthesise Modulo %d\nStyle=%s', value, style);  style=Scheduled  visibilities=1024+32768  constraintInUse=off  constraintRelation=>  constraintLimit=2  version=20090407
  q : Outport
  qv : Outport  Port=2
  qc : Outport  Port=3
  wires:
  av/1 -> ChannelIn/1
  ac/1 -> ChannelIn/2
  a/1 -> ChannelIn/3
  sin/1 -> ChannelIn/4
  cos/1 -> ChannelIn/5
  ChannelIn/3 -> QxSin/2, Add_I_Reg1/1  "inQ"
  ChannelIn/4 -> QxSin/1
  ChannelIn/5 -> IxCos/1
  ChannelOut/1 -> qv/1
  ChannelOut/2 -> qc/1
  ChannelOut/3 -> q/1
  Sub/1 -> ChannelOut/3
  ChannelIn/2 -> BitExtract1/1
  Const2/1 -> Channel_1/2
  BitExtract1/1 -> Channel_1/1
  Channel_1/1 -> And1/2
  Add_I_Reg1/1 -> IxCos/2  "inI"
  ChannelIn/1 -> And1/1
  And1/1 -> Delay2/1
  Delay2/1 -> ChannelOut/1
  Const3/1 -> ChannelOut/2
  IxCos/1 -> Sub/1
  QxSin/1 -> Sub/2

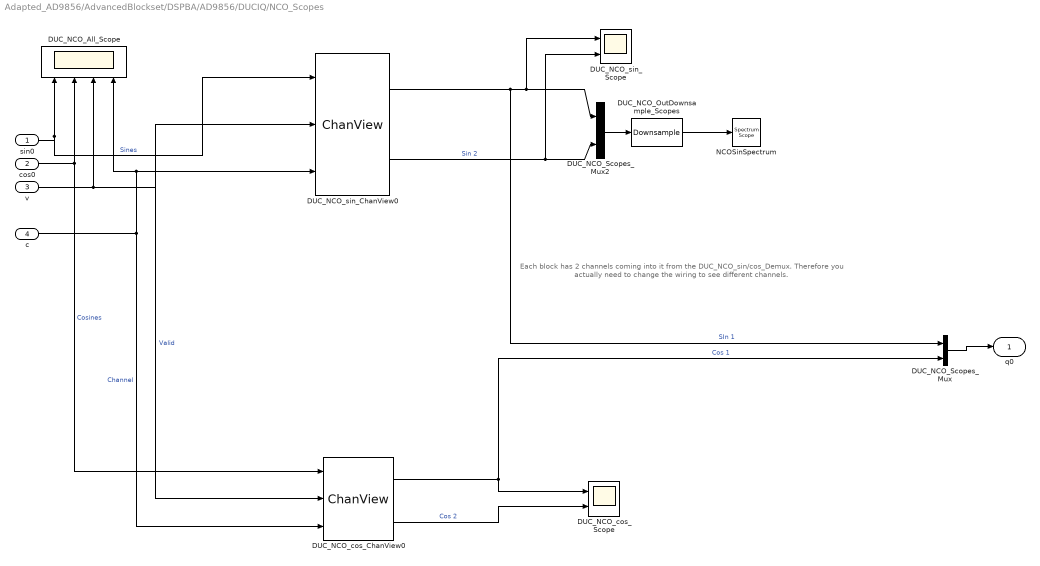
== system Adapted_AD9856/AdvancedBlockset/DSPBA/AD9856/DUCIQ/NCO_Scopes ==
  note: Each block has 2 channels
      | coming into it from the DUC_NCO_sin/cos_Demux. Therefore
      | you actually need to change the wiring to see different channels.
  sin0 : Inport
  cos0 : Inport  Port=2
  v : Inport  Port=3
  c : Inport  Port=4
  DUC_NCO_All_Scope : Scope  NumInputPorts=4
      settings: TimeRange=10000  YMin=-1~0~0~-5  YMax=1~1~15~5  SaveName=ScopeData29
  DUC_NCO_OutDownsample_Scopes : dspsigops/Downsample  N=2  phase=0  InputProcessing=Inherited (this choice will be removed - see release notes)  RateOptions=Enforce single-rate processing  smode=Allow multirate  fmode=Maintain input frame size  ic=0
  DUC_NCO_Scopes_Mux : Mux  Inputs=2
  DUC_NCO_Scopes_Mux2 : Mux  Inputs=2
  DUC_NCO_cos_ChanView0 : DSPBABase/ChanView  nchans=2  chan_vector=[0 1]  outsvalid=off  latency=2  version=20090407
  DUC_NCO_cos_Scope : Scope  NumInputPorts=2
      settings: TimeRange=10000  YMin=-1~-1  YMax=1~1  SaveName=ScopeData3
  DUC_NCO_sin_ChanView0 : DSPBABase/ChanView  nchans=2  chan_vector=[0:1]  outsvalid=off  latency=2  version=20090407
  DUC_NCO_sin_Scope : Scope  NumInputPorts=2
      settings: TimeRange=10000  YMin=-1~-1  YMax=1~1  SaveName=ScopeData6
  NCOSinSpectrum : dspsnks4/Spectrum Scope  DialogController=dspdialog.SpectrumScope  DialogControllerArgs=DataTag1  SystemSampleTime=-1  ScopeProperties=on  Domain=Frequency  HorizSpan=1  UseBuffer=on  BufferSize=4096  Overlap=0  inpFftLenInherit=off  FFTlength=128  numAvg=1  DisplayProperties=off  AxisGrid=on  Memory=off  FrameNumber=on  AxisLegend=on  AxisZoom=off  OpenScopeAtSimStart=off  OpenScopeImmediately=off  FigPos=get(0,'defaultfigureposition')  AxisProperties=off  XUnits=Hertz  XRange=[0...Fs/2]  XDisplay=0  InheritXIncr=off  XIncr=1/(100e6)  XLabel=Samples  XLimit=Auto  YUnits=dB  XMax=1  XMin=0  YLabel=Magnitude-squared, dB  LineProperties=off  LineDisables=on|on|on|on|on|on|on  LineStyles=-  LineMarkers=None  LineColors=[1 0 1]|[0 0 1]|[1 0 0]|[0 1 0]|[0 1 1]||[1 1 0]|[1 0 0]  wintypeSpecScope=Hann  RsSpecScope=50  betaSpecScope=5  winsampSpecScope=Periodic  XAxisParamsVer=6.8
      settings: YMin=-114.271541020359  YMax=31.1780270467433
  q0 : Outport
  wires:
  sin0/1 -> DUC_NCO_All_Scope/1, DUC_NCO_sin_ChanView0/1  "Sines"
  c/1 -> DUC_NCO_sin_ChanView0/3, DUC_NCO_All_Scope/4, DUC_NCO_cos_ChanView0/3  "Channel"
  v/1 -> DUC_NCO_sin_ChanView0/2, DUC_NCO_cos_ChanView0/2, DUC_NCO_All_Scope/3  "Valid"
  cos0/1 -> DUC_NCO_All_Scope/2, DUC_NCO_cos_ChanView0/1  "Cosines"
  DUC_NCO_sin_ChanView0/1 -> DUC_NCO_Scopes_Mux/1, DUC_NCO_Scopes_Mux2/1, DUC_NCO_sin_Scope/1  "SIn 1"
  DUC_NCO_sin_ChanView0/2 -> DUC_NCO_Scopes_Mux2/2, DUC_NCO_sin_Scope/2  "Sin 2"
  DUC_NCO_cos_ChanView0/1 -> DUC_NCO_cos_Scope/1, DUC_NCO_Scopes_Mux/2  "Cos 1"
  DUC_NCO_cos_ChanView0/2 -> DUC_NCO_cos_Scope/2  "Cos 2"
  DUC_NCO_Scopes_Mux/1 -> q0/1
  DUC_NCO_OutDownsample_Scopes/1 -> NCOSinSpectrum/1
  DUC_NCO_Scopes_Mux2/1 -> DUC_NCO_OutDownsample_Scopes/1
